simulink model "multibody"  (R2025b)
settings: Solver=ode45  StartTime=0.0  StopTime=250  RelTol=1e-3  AbsTol=1e-3  EnableMultiTasking=on
undefined symbols (not defined in the file or in its folder): X, Y, Z
libraries: sm_lib x11, nesl_utility x7, simulink x2
settings Model: Creator=mrrom  LastModifiedBy=mrrom
settings SolverCC: AutoScaleAbsTol=off  AlgebraicLoopSolver=TrustRegion  MaxZcPerStep=1.0
settings DataIOCC: LimitDataPoints=on  MaxDataPoints=10000
settings OptimizationCC: ReuseModelBlockBuffer=off  LifeSpan=inf
settings DebuggingCC: UnconnectedInputMsg=warning  UnconnectedOutputMsg=warning  UnconnectedLineMsg=warning  AllowSymbolicDim=off  SubsystemReferenceDiagnosticForUnitTest=warning  SFUnexpectedBacktrackingDiag=warning  SFNoUnconditionalDefaultTransitionDiag=warning  SFExecutionAtInitializationDiag=none  ArithmeticOperatorsInVariantConditions=warning
settings ModelReferenceCC: EnableRefExpFcnMdlSchedulingChecks=on
settings SFSimCC: SimUseLocalCustomCode=off  CustomCodeUndefinedFunction=UseInterfaceOnly
settings RTWCC: RTWUseLocalCustomCode=off  GPUComputeCapability=3.5  DLArmComputeVersion=19.05
settings CodeAppCC: StateflowObjectComments=on
settings GRTTargetCC: TargetLangStandard=C89/C90 (ANSI)
settings ConfigComp: CovMetricSettings=dw  CovSaveCumulativeToWorkspaceVar=on  CovSaveSingleToWorkspaceVar=on  CovExternalEMLEnable=off  CovSFcnEnable=off
settings SimscapeCC: SimscapeLogType=all  SimscapeLogSimulationStatistics=on  SimscapeLogDataHistory=10000.0

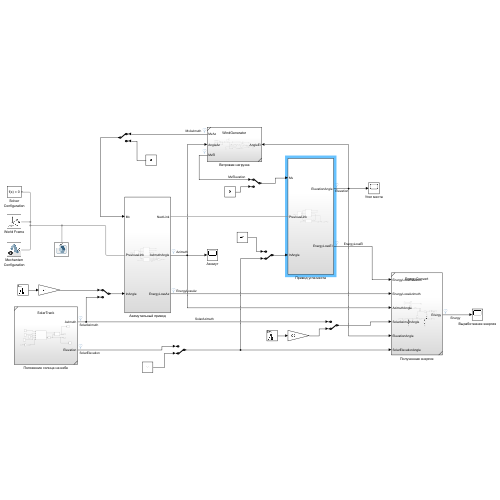
[thumbnail: Simulink's stored preview of the top-level diagram]
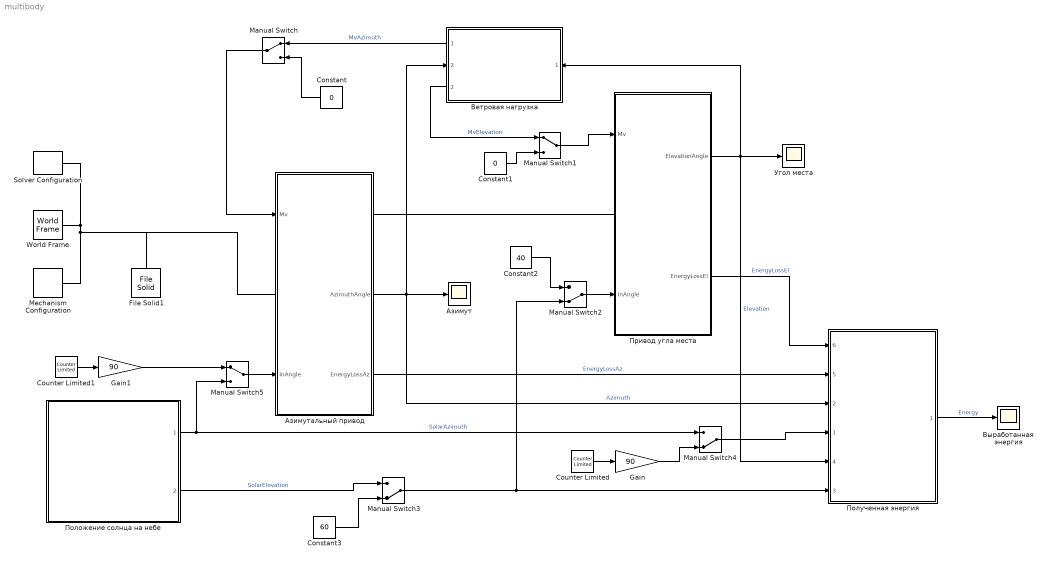
== system multibody ==
  Constant : Constant  Value=0
  Constant1 : Constant  Value=0
  Constant2 : Constant  Value=40
  Constant3 : Constant  Value=60
  Counter Limited : simulink/Sources/Counter Limited  uplimit=24  tsamp=12
  Counter Limited1 : simulink/Sources/Counter Limited  uplimit=24  tsamp=12
  File Solid1 : sm_lib/Body Elements/File Solid  ExtGeomFileName=.\3dmodel\основание.STEP  UnitType=FromFile  ExtGeomFileUnits=m  StepReaderType=HEX  ExportConvexHullGeometry=off  InertiaType=Custom  BasedOnType=DensityFromFile  Density=1000  DensityUnits=kg/m^3  Mass=937  MassUnits=kg  CenterOfMass=[0 0 0.03]  CenterOfMassUnits=m  MomentsOfInertia=[179.75 179.75 359.1]  MomentsOfInertiaUnits=kg*m^2  ProductsOfInertia=[0 0 0]  ProductsOfInertiaUnits=kg*m^2  GraphicType=FromGeometry  MarkerShape=Sphere  MarkerSize=10  GraphicVisPropType=SimpleVisualProperties  GraphicDiffuseColor=[0.5 0.5 0.5]  GraphicOpacity=1.0  GraphicSpecularColor=[0.5 0.5 0.5 1.0]  GraphicAmbientColor=[0.15 0.15 0.15 1.0]  GraphicEmissiveColor=[0.0 0.0 0.0 1.0]  GraphicShininess=75  DoExposeReferenceFrame=on  SerializedFrames=<Frames/>
  Gain : Gain  Gain=90
  Gain1 : Gain  Gain=90
  Manual Switch : ManualSwitch
  Manual Switch1 : ManualSwitch
  Manual Switch2 : ManualSwitch  CurrentSetting=0
  Manual Switch3 : ManualSwitch  CurrentSetting=0
  Manual Switch4 : ManualSwitch  CurrentSetting=0
  Manual Switch5 : ManualSwitch
  Mechanism Configuration : sm_lib/Utilities/Mechanism Configuration  UniformGravity=Constant  GravityVector=[0 0 -9.80665]  GravityVectorUnits=m/s^2  LinearizationDelta=0.001  JointModeTransitionNonlinearIterations=2
  Solver Configuration : nesl_utility/Solver Configuration  PhysicalDomain=network_engine_domain  SubClassName=solver  LeftPortType=input  RightPortType=generic  Tones=[]  Harmonics=[]  SimulateNoise=off  Profile=off  UseLocalSampling=off  EnableSwitchedLinearOptims=on  FrequencyDomain=off  UseCCode=off  RelTol=0.001  AbsTol=1e-06  MinStep=1e-09  ToWorkspace=off  RevertToSquareIcSolve=off  NumHomotopyIterations=100  PhasorMode=off  PhasorModeNumHarmonics=1  ConsistencySolver=NEWTON_XTOL_AFTER_FTOL  IndexReductionMethod=DerivativeReplacement  DoDC=off  ResidualTolerance=1e-09  ConsistencyTolSource=GLOBAL  ConsistencyAbsTol=0.001  ConsistencyRelTol=0.001  ConsistencyTolFactor=0.001  UseLocalSolver=off  LocalSolverChoice=NE_BACKWARD_EULER_ADVANCER  ResolveIndetEquations=on  FunctionEvalNumThread=1  LocalSolverSampleTime=0.001  DoFixedCost=off  MaxNonlinIter=3  MaxModeIter=2  ComputeImpulses=off  ImpulseIterations=2  LinearAlgebra=Sparse  LinearAlgebraNumThread=0  EquationFormulation=NE_TIME_EF  DelaysMemoryBudget=1024  AutomaticFiltering=on  FilteringTimeConstant=0.001  PartitionStorageMethod=AS_NEEDED  PartitionMemoryBudget=1024  PartitionMethod=FAST  MultibodyUseLocalSolver=off  MultibodyLocalSolverChoice=ODE1  MultibodyLocalSolverSampleTime=0.001
  World Frame : sm_lib/Frames and Transforms/World Frame
  Азимут : Scope
      settings: ActiveDisplayYMinimum=-57.83463  ActiveDisplayYMaximum=57.51622  DataLoggingVariableName=ScopeData2
  Азимутальный привод : Subsystem
      settings: PortSchema="{\"entries\":[{\"content\":{\"sides\":[{\"content\":{\"connectorIds\":[\"In1\",\"LConn1\",\"In2\"]},\"type\":\"ConnectorPlacement.EquallySpacedRectSide\",\"uuid\":\"74c85136-bb4f-42ec-9268-4578d06108e1\"},{\"content\":{\"connectorIds\":[\"RConn1\",\"Out1\",\"Out2\"],\"side\":\"RIGHT\"},\"type\":\"ConnectorPlacement.EquallySpacedRectSide\",\"uuid\":\"6853e412-fedd-4b61-b862-224afc6f9efb\"},{\"content\":{\"side\":\"TOP\"},\"type\":\"ConnectorPlacement.EquallySpacedRectSide\",\"uuid\":\"9a3f1114-26e6-4ebe-9104-1c58e9eb491f\"}]},\"type\":\"ConnectorPlacement.EquallySpacedConnector\",\"uuid\":\"8bfaaf63-3e5e-4e48-8a8c-615e04096f38\"}],\"packageUris\":[\"http://schema.mathworks.com/mf0/Connector/R2020b\"],\"version\":\"1.0\"}"
  Ветровая нагрузка : Subsystem  ReferencedSubsystem=WindGenerator
      settings: PortSchema="{\"entries\":[{\"content\":{\"sides\":[{\"content\":{\"connectorIds\":[\"In1\"]},\"type\":\"ConnectorPlacement.EquallySpacedRectSide\",\"uuid\":\"4795a72d-e259-4e5d-912f-69a3ba47a917\"},{\"content\":{\"connectorIds\":[\"Out1\",\"In2\",\"Out2\"],\"side\":\"RIGHT\"},\"type\":\"ConnectorPlacement.EquallySpacedRectSide\",\"uuid\":\"787660c0-9a7a-4bf4-8302-266ce8ff8086\"},{\"content\":{\"side\":\"TOP\"},\"type\":\"ConnectorPlacement.EquallySpacedRectSide\",\"uuid\":\"a4e869d2-b73f-459f-85e5-790c0c0164f4\"}]},\"type\":\"ConnectorPlacement.EquallySpacedConnector\",\"uuid\":\"c4a08e61-f882-4463-a797-212d49c9ab89\"}],\"packageUris\":[\"http://schema.mathworks.com/mf0/Connector/R2020b\"],\"version\":\"1.0\"}"
  Выработанная энергия : Scope
      settings: ActiveDisplayYMinimum=-4298.79553  ActiveDisplayYMaximum=38689.15976  DataLoggingVariableName=ScopeData4
  Положение солнца на небе : Subsystem  ReferencedSubsystem=SolarTrack
  Полученная энергия : Subsystem  ReferencedSubsystem=EnergyConvert
      settings: PortSchema="{\"entries\":[{\"content\":{\"sides\":[{\"content\":{\"connectorIds\":[\"In6\",\"In5\",\"In2\",\"In1\",\"In4\",\"In3\"]},\"type\":\"ConnectorPlacement.EquallySpacedRectSide\",\"uuid\":\"6662d747-a41b-4524-af57-34fa7ccd50e7\"},{\"content\":{\"connectorIds\":[\"Out1\"],\"side\":\"RIGHT\"},\"type\":\"ConnectorPlacement.EquallySpacedRectSide\",\"uuid\":\"fbbb3776-687f-4ce7-b440-113aef165e6d\"},{\"content\":{\"side\":\"TOP\"},\"type\":\"ConnectorPlacement.EquallySpacedRectSide\",\"uuid\":\"61cd8f2a-a046-4d6d-8da3-a48999f51fae\"}]},\"type\":\"ConnectorPlacement.EquallySpacedConnector\",\"uuid\":\"39e6c406-5663-4613-aeb7-dacef6da2c4e\"}],\"packageUris\":[\"http://schema.mathworks.com/mf0/Connector/R2020b\"],\"version\":\"1.0\"}"
  Привод угла места : Subsystem
      settings: PortSchema="{\"entries\":[{\"content\":{\"sides\":[{\"content\":{\"connectorIds\":[\"In1\",\"LConn1\",\"In2\"]},\"type\":\"ConnectorPlacement.EquallySpacedRectSide\",\"uuid\":\"dffe733f-0464-4532-825b-a2634fb65552\"},{\"content\":{\"connectorIds\":[\"Out1\",\"Out2\"],\"side\":\"RIGHT\"},\"type\":\"ConnectorPlacement.EquallySpacedRectSide\",\"uuid\":\"657db495-a866-4286-af61-dacf0e8f46cf\"},{\"content\":{\"side\":\"TOP\"},\"type\":\"ConnectorPlacement.EquallySpacedRectSide\",\"uuid\":\"2facb6e5-1fba-4ec7-9e73-47f303272759\"}]},\"type\":\"ConnectorPlacement.EquallySpacedConnector\",\"uuid\":\"76ec8b90-f482-44a4-b7c8-1753a66156a3\"}],\"packageUris\":[\"http://schema.mathworks.com/mf0/Connector/R2020b\"],\"version\":\"1.0\"}"
  Угол места : Scope
      settings: ActiveDisplayYMinimum=-7.64121  ActiveDisplayYMaximum=68.76786  DataLoggingVariableName=ScopeData3
  wires:
  Привод угла места/1(ElevationAngle) -> Полученная энергия/4, Угол места/1, Ветровая нагрузка/1  "Elevation"
  Азимутальный привод/1(AzimuthAngle) -> Ветровая нагрузка/2, Азимут/1, Полученная энергия/2  "Azimuth"
  Положение солнца на небе/2 -> Manual Switch3/1  "SolarElevation"
  Положение солнца на небе/1 -> Manual Switch4/1, Manual Switch5/2  "SolarAzimuth"
  Азимутальный привод/2(EnergyLossAz) -> Полученная энергия/5  "EnergyLossAz"
  Привод угла места/2(EnergyLossEl) -> Полученная энергия/6  "EnergyLossEl"
  Ветровая нагрузка/2 -> Manual Switch1/1  "MvElevation"
  Ветровая нагрузка/1 -> Manual Switch/1  "MvAzimuth"
  Полученная энергия/1 -> Выработанная энергия/1  "Energy"
  Constant/1 -> Manual Switch/2
  Manual Switch/1 -> Азимутальный привод/1(Mv)
  Constant1/1 -> Manual Switch1/2
  Manual Switch1/1 -> Привод угла места/1(Mv)
  Manual Switch2/1 -> Привод угла места/2(InAngle)
  Constant2/1 -> Manual Switch2/1
  Constant3/1 -> Manual Switch3/2
  Counter Limited/1 -> Gain/1
  Gain/1 -> Manual Switch4/2
  Manual Switch4/1 -> Полученная энергия/1
  Counter Limited1/1 -> Gain1/1
  Gain1/1 -> Manual Switch5/1
  Manual Switch5/1 -> Азимутальный привод/2(InAngle)
  Manual Switch3/1 -> Manual Switch2/2, Полученная энергия/3
  connections:
  World Frame/RConn1 -- File Solid1/RConn1 -- Азимутальный привод/LConn1 -- Mechanism Configuration/RConn1 -- Solver Configuration/RConn1
  Азимутальный привод/RConn1 -- Привод угла места/LConn1

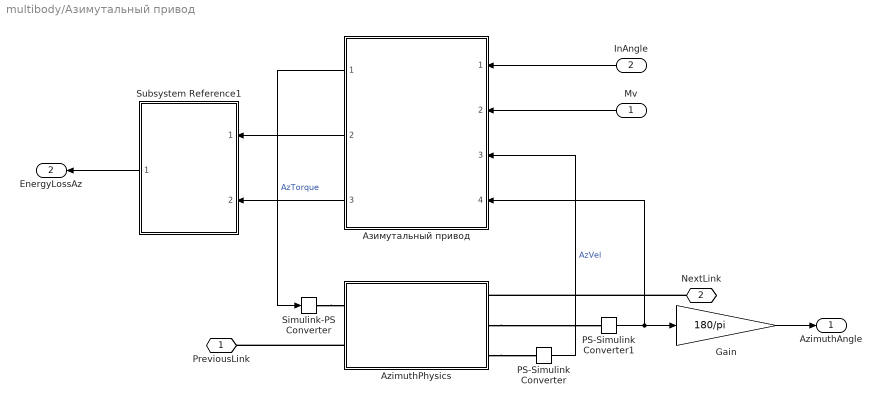
== system multibody/Азимутальный привод ==
  Mv : Inport
  InAngle : Inport  Port=2
  AzimuthPhysics : Subsystem
  Gain : Gain  Gain=180/pi
  PS-Simulink Converter : nesl_utility/PS-Simulink Converter  PhysicalDomain=network_engine_domain  SubClassName=ps_output  LeftPortType=input  RightPortType=output  PseudoPeriodic=off  Frequencies=[]  VectorFormat=inherit  Unit=inherit  AffineConversion=off
  PS-Simulink Converter1 : nesl_utility/PS-Simulink Converter  PhysicalDomain=network_engine_domain  SubClassName=ps_output  LeftPortType=input  RightPortType=output  PseudoPeriodic=off  Frequencies=[]  VectorFormat=inherit  Unit=inherit  AffineConversion=off
  Simulink-PS Converter : nesl_utility/Simulink-PS Converter  PhysicalDomain=network_engine_domain  SubClassName=ps_input  LeftPortType=input  RightPortType=output  PseudoPeriodic=off  Frequencies=[]  NoiseDistribution=none  NoiseParameters=[]  Unit=1  AffineConversion=off  FilteringAndDerivatives=provide  SimscapeFilterOrder=1  InputFilterTimeConstant=0.001  UdotUserProvided=0
  Subsystem Reference1 : Subsystem  ReferencedSubsystem=MotorEnergyLoss
  Азимутальный привод : Subsystem  ReferencedSubsystem=Actuator
  PreviousLink : PMIOPort  Side=Left
  NextLink : PMIOPort  Port=2  Side=Right
  AzimuthAngle : Outport
  EnergyLossAz : Outport  Port=2
  wires:
  PS-Simulink Converter/1 -> Азимутальный привод/3  "AzVel"
  Азимутальный привод/1 -> Simulink-PS Converter/1  "AzTorque"
  InAngle/1 -> Азимутальный привод/1
  Mv/1 -> Азимутальный привод/2
  Gain/1 -> AzimuthAngle/1
  PS-Simulink Converter1/1 -> Gain/1, Азимутальный привод/4
  Азимутальный привод/2 -> Subsystem Reference1/1
  Азимутальный привод/3 -> Subsystem Reference1/2
  Subsystem Reference1/1 -> EnergyLossAz/1
  connections:
  AzimuthPhysics/RConn3 -- PS-Simulink Converter/LConn1
  NextLink/RConn1 -- AzimuthPhysics/RConn1
  AzimuthPhysics/LConn2 -- PreviousLink/RConn1
  Simulink-PS Converter/RConn1 -- AzimuthPhysics/LConn1
  AzimuthPhysics/RConn2 -- PS-Simulink Converter1/LConn1

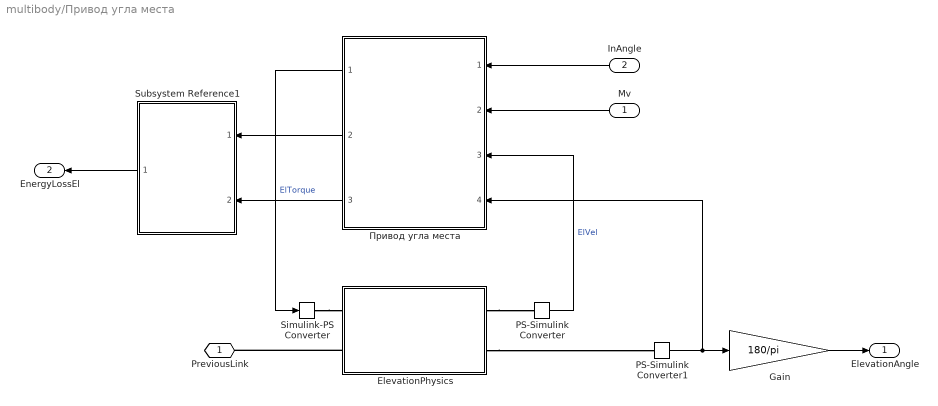
== system multibody/Привод угла места ==
  Mv : Inport
  InAngle : Inport  Port=2
  ElevationPhysics : Subsystem
  Gain : Gain  Gain=180/pi
  PS-Simulink Converter : nesl_utility/PS-Simulink Converter  PhysicalDomain=network_engine_domain  SubClassName=ps_output  LeftPortType=input  RightPortType=output  PseudoPeriodic=off  Frequencies=[]  VectorFormat=inherit  Unit=inherit  AffineConversion=off
  PS-Simulink Converter1 : nesl_utility/PS-Simulink Converter  PhysicalDomain=network_engine_domain  SubClassName=ps_output  LeftPortType=input  RightPortType=output  PseudoPeriodic=off  Frequencies=[]  VectorFormat=inherit  Unit=inherit  AffineConversion=off
  Simulink-PS Converter : nesl_utility/Simulink-PS Converter  PhysicalDomain=network_engine_domain  SubClassName=ps_input  LeftPortType=input  RightPortType=output  PseudoPeriodic=off  Frequencies=[]  NoiseDistribution=none  NoiseParameters=[]  Unit=1  AffineConversion=off  FilteringAndDerivatives=provide  SimscapeFilterOrder=1  InputFilterTimeConstant=0.001  UdotUserProvided=0
  Subsystem Reference1 : Subsystem  ReferencedSubsystem=MotorEnergyLoss
  Привод угла места : Subsystem  ReferencedSubsystem=Actuator
  PreviousLink : PMIOPort  Side=Left
  ElevationAngle : Outport
  EnergyLossEl : Outport  Port=2
  wires:
  InAngle/1 -> Привод угла места/1
  Mv/1 -> Привод угла места/2
  PS-Simulink Converter/1 -> Привод угла места/3  "ElVel"
  Привод угла места/1 -> Simulink-PS Converter/1  "ElTorque"
  Gain/1 -> ElevationAngle/1
  PS-Simulink Converter1/1 -> Привод угла места/4, Gain/1
  Привод угла места/2 -> Subsystem Reference1/1
  Subsystem Reference1/1 -> EnergyLossEl/1
  Привод угла места/3 -> Subsystem Reference1/2
  connections:
  ElevationPhysics/RConn1 -- PS-Simulink Converter/LConn1
  ElevationPhysics/LConn2 -- PreviousLink/RConn1
  Simulink-PS Converter/RConn1 -- ElevationPhysics/LConn1
  ElevationPhysics/RConn2 -- PS-Simulink Converter1/LConn1

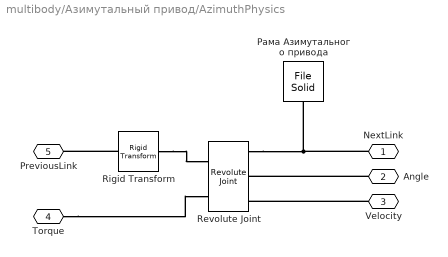
== system multibody/Азимутальный привод/AzimuthPhysics ==
  Revolute Joint : sm_lib/Joints/Revolute Joint  JointMode=Normal  CompositeWrenchDir=FollowerOnBase  CompositeWrenchFrame=BaseFrame  SenseConstraintForce=off  SenseConstraintTorque=off  SenseTotalForce=off  SenseTotalTorque=off  PositionTargetSpecify=off  PositionTargetPriority=High  PositionTargetValue=0  PositionTargetValueUnits=deg  VelocityTargetSpecify=off  VelocityTargetPriority=High  VelocityTargetValue=0  VelocityTargetValueUnits=deg/s  EquilibriumPosition=0  EquilibriumPositionUnits=deg  SpringStiffness=0  SpringStiffnessUnits=N*m/deg  DampingCoefficient=0  DampingCoefficientUnits=N*m/(deg/s)  LowerLimitSpecify=off  LowerLimitBound=-90  LowerLimitBoundUnits=deg  LowerLimitStiffness=1e4  LowerLimitStiffnessUnits=N*m/deg  LowerLimitDamping=10  LowerLimitDampingUnits=N*m/(deg/s)  LowerLimitTransitionRegionWidth=0.1  LowerLimitTransitionRegionWidthUnits=deg  UpperLimitSpecify=off  UpperLimitBound=90  UpperLimitBoundUnits=deg  UpperLimitStiffness=1e4  UpperLimitStiffnessUnits=N*m/deg  UpperLimitDamping=10  UpperLimitDampingUnits=N*m/(deg/s)  UpperLimitTransitionRegionWidth=0.1  UpperLimitTransitionRegionWidthUnits=deg  TorqueActuationMode=InputTorque  MotionActuationMode=ComputedMotion  SensePosition=on  SenseVelocity=on  SenseAcceleration=off  SenseTorqueForce=off  SenseLowerLimitTorqueForce=off  SenseUpperLimitTorqueForce=off
  Rigid Transform : sm_lib/Frames and Transforms/Rigid Transform  RotationMethod=None  FollAlignAxisA=+X  BaseAlignAxisA=+Y  FollAlignAxisB=+Y  BaseAlignAxisB=+Z  RotationStandardAxis=+Z  RotationAngle=0  RotationAngleUnits=deg  RotationArbitraryAxis=[0 0 1]  RotationSequenceAxes=FollowerAxes  RotationSequence=XYX  RotationSequenceAngles=[0 0 0]  RotationSequenceAnglesUnits=deg  RotationMatrix=[1 0 0; 0 1 0; 0 0 1]  Quaternion=[1 0 0 0]  TranslationMethod=None  TranslationCartesianOffset=[0 0 0]  TranslationCartesianOffsetUnits=m  TranslationStandardAxis=+Z  TranslationStandardOffset=0  TranslationStandardOffsetUnits=m  TranslationROffset=0  TranslationROffsetUnits=m  TranslationThetaOffset=0  TranslationThetaOffsetUnits=deg  TranslationZOffset=0  TranslationZOffsetUnits=m
  Рама Азимутального привода : sm_lib/Body Elements/File Solid  ExtGeomFileName=.\3dmodel\Рама.STEP  UnitType=FromFile  ExtGeomFileUnits=m  StepReaderType=HEX  ExportConvexHullGeometry=off  InertiaType=Custom  BasedOnType=DensityFromFile  Density=1000  DensityUnits=kg/m^3  Mass=23.33  MassUnits=kg  CenterOfMass=[0 0 0.29]  CenterOfMassUnits=m  MomentsOfInertia=[1.54 12.25 10.72]  MomentsOfInertiaUnits=kg*m^2  ProductsOfInertia=[0 0 0]  ProductsOfInertiaUnits=kg*m^2  GraphicType=FromGeometry  MarkerShape=Sphere  MarkerSize=10  GraphicVisPropType=SimpleVisualProperties  GraphicDiffuseColor=[0.5 0.5 0.5]  GraphicOpacity=1.0  GraphicSpecularColor=[0.5 0.5 0.5 1.0]  GraphicAmbientColor=[0.15 0.15 0.15 1.0]  GraphicEmissiveColor=[0.0 0.0 0.0 1.0]  GraphicShininess=75  DoExposeReferenceFrame=on  SerializedFrames=<Frames/>
  NextLink : PMIOPort  Side=Right
  Angle : PMIOPort  Port=2  Side=Right
  Velocity : PMIOPort  Port=3  Side=Right
  Torque : PMIOPort  Port=4  Side=Left
  PreviousLink : PMIOPort  Port=5  Side=Left
  connections:
  Velocity/RConn1 -- Revolute Joint/RConn3
  Torque/RConn1 -- Revolute Joint/LConn2
  Revolute Joint/RConn1 -- NextLink/RConn1 -- Рама Азимутального привода/RConn1
  Rigid Transform/LConn1 -- PreviousLink/RConn1
  Angle/RConn1 -- Revolute Joint/RConn2
  Rigid Transform/RConn1 -- Revolute Joint/LConn1

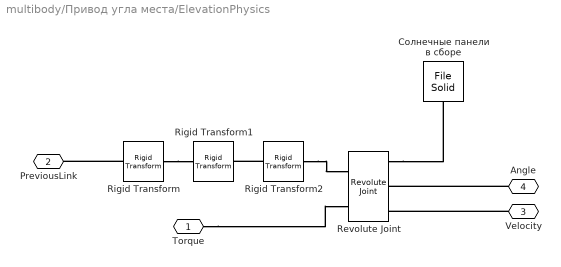
== system multibody/Привод угла места/ElevationPhysics ==
  Revolute Joint : sm_lib/Joints/Revolute Joint  JointMode=Normal  CompositeWrenchDir=FollowerOnBase  CompositeWrenchFrame=BaseFrame  SenseConstraintForce=off  SenseConstraintTorque=off  SenseTotalForce=off  SenseTotalTorque=off  PositionTargetSpecify=off  PositionTargetPriority=High  PositionTargetValue=0  PositionTargetValueUnits=deg  VelocityTargetSpecify=off  VelocityTargetPriority=High  VelocityTargetValue=0  VelocityTargetValueUnits=deg/s  EquilibriumPosition=0  EquilibriumPositionUnits=deg  SpringStiffness=0  SpringStiffnessUnits=N*m/deg  DampingCoefficient=0  DampingCoefficientUnits=N*m/(deg/s)  LowerLimitSpecify=off  LowerLimitBound=-90  LowerLimitBoundUnits=deg  LowerLimitStiffness=1e4  LowerLimitStiffnessUnits=N*m/deg  LowerLimitDamping=10  LowerLimitDampingUnits=N*m/(deg/s)  LowerLimitTransitionRegionWidth=0.1  LowerLimitTransitionRegionWidthUnits=deg  UpperLimitSpecify=off  UpperLimitBound=90  UpperLimitBoundUnits=deg  UpperLimitStiffness=1e4  UpperLimitStiffnessUnits=N*m/deg  UpperLimitDamping=10  UpperLimitDampingUnits=N*m/(deg/s)  UpperLimitTransitionRegionWidth=0.1  UpperLimitTransitionRegionWidthUnits=deg  TorqueActuationMode=InputTorque  MotionActuationMode=ComputedMotion  SensePosition=on  SenseVelocity=on  SenseAcceleration=off  SenseTorqueForce=off  SenseLowerLimitTorqueForce=off  SenseUpperLimitTorqueForce=off
  Rigid Transform : sm_lib/Frames and Transforms/Rigid Transform  RotationMethod=StandardAxis  FollAlignAxisA=+X  BaseAlignAxisA=+Y  FollAlignAxisB=+Y  BaseAlignAxisB=+Z  RotationStandardAxis=+X  RotationAngle=90  RotationAngleUnits=deg  RotationArbitraryAxis=[0 0 1]  RotationSequenceAxes=FollowerAxes  RotationSequence=XYX  RotationSequenceAngles=[0 0 0]  RotationSequenceAnglesUnits=deg  RotationMatrix=[1 0 0; 0 1 0; 0 0 1]  Quaternion=[1 0 0 0]  TranslationMethod=StandardAxis  TranslationCartesianOffset=[0 0 0]  TranslationCartesianOffsetUnits=m  TranslationStandardAxis=+Z  TranslationStandardOffset=893  TranslationStandardOffsetUnits=mm  TranslationROffset=0  TranslationROffsetUnits=m  TranslationThetaOffset=0  TranslationThetaOffsetUnits=deg  TranslationZOffset=0  TranslationZOffsetUnits=m
  Rigid Transform1 : sm_lib/Frames and Transforms/Rigid Transform  RotationMethod=StandardAxis  FollAlignAxisA=+X  BaseAlignAxisA=+Y  FollAlignAxisB=+Y  BaseAlignAxisB=+Z  RotationStandardAxis=+Y  RotationAngle=90  RotationAngleUnits=deg  RotationArbitraryAxis=[0 0 1]  RotationSequenceAxes=FollowerAxes  RotationSequence=XYX  RotationSequenceAngles=[0 0 0]  RotationSequenceAnglesUnits=deg  RotationMatrix=[1 0 0; 0 1 0; 0 0 1]  Quaternion=[1 0 0 0]  TranslationMethod=None  TranslationCartesianOffset=[0 0 0]  TranslationCartesianOffsetUnits=m  TranslationStandardAxis=+Z  TranslationStandardOffset=893  TranslationStandardOffsetUnits=mm  TranslationROffset=0  TranslationROffsetUnits=m  TranslationThetaOffset=0  TranslationThetaOffsetUnits=deg  TranslationZOffset=0  TranslationZOffsetUnits=m
  Rigid Transform2 : sm_lib/Frames and Transforms/Rigid Transform  RotationMethod=StandardAxis  FollAlignAxisA=+X  BaseAlignAxisA=+Y  FollAlignAxisB=+Y  BaseAlignAxisB=+Z  RotationStandardAxis=+Z  RotationAngle=-90  RotationAngleUnits=deg  RotationArbitraryAxis=[0 0 1]  RotationSequenceAxes=FollowerAxes  RotationSequence=XYX  RotationSequenceAngles=[0 0 0]  RotationSequenceAnglesUnits=deg  RotationMatrix=[1 0 0; 0 1 0; 0 0 1]  Quaternion=[1 0 0 0]  TranslationMethod=None  TranslationCartesianOffset=[0 0 0]  TranslationCartesianOffsetUnits=m  TranslationStandardAxis=+Z  TranslationStandardOffset=893  TranslationStandardOffsetUnits=mm  TranslationROffset=0  TranslationROffsetUnits=m  TranslationThetaOffset=0  TranslationThetaOffsetUnits=deg  TranslationZOffset=0  TranslationZOffsetUnits=m
  Солнечные панели в сборе : sm_lib/Body Elements/File Solid  ExtGeomFileName=.\3dmodel\сборкасбласт.STEP  UnitType=FromFile  ExtGeomFileUnits=m  StepReaderType=HEX  ExportConvexHullGeometry=off  InertiaType=Custom  BasedOnType=DensityFromFile  Density=1000  DensityUnits=kg/m^3  Mass=38.55  MassUnits=kg  CenterOfMass=[-0.03 0 0]  CenterOfMassUnits=m  MomentsOfInertia=[8.53 15.23 6.71]  MomentsOfInertiaUnits=kg*m^2  ProductsOfInertia=[0 0 0]  ProductsOfInertiaUnits=kg*m^2  GraphicType=FromGeometry  MarkerShape=Sphere  MarkerSize=10  GraphicVisPropType=SimpleVisualProperties  GraphicDiffuseColor=[0.5 0.5 0.5]  GraphicOpacity=1.0  GraphicSpecularColor=[0.5 0.5 0.5 1.0]  GraphicAmbientColor=[0.15 0.15 0.15 1.0]  GraphicEmissiveColor=[0.0 0.0 0.0 1.0]  GraphicShininess=75  DoExposeReferenceFrame=on  SerializedFrames=<Frames/>
  Torque : PMIOPort  Side=Left
  PreviousLink : PMIOPort  Port=2  Side=Left
  Velocity : PMIOPort  Port=3  Side=Right
  Angle : PMIOPort  Port=4  Side=Right
  connections:
  Velocity/RConn1 -- Revolute Joint/RConn3
  Torque/RConn1 -- Revolute Joint/LConn2
  Revolute Joint/RConn1 -- Солнечные панели в сборе/RConn1
  Rigid Transform/LConn1 -- PreviousLink/RConn1
  Angle/RConn1 -- Revolute Joint/RConn2
  Rigid Transform/RConn1 -- Rigid Transform1/LConn1
  Rigid Transform2/LConn1 -- Rigid Transform1/RConn1
  Rigid Transform2/RConn1 -- Revolute Joint/LConn1
